simulink model "A10_DC_Motor_Antriebsstrang"  (R2017b)
settings: Solver=ode45  StartTime=0.0  StopTime=10  MaxStep=1E-3  RelTol=1e-3  EnableMultiTasking=on
values from neighbouring files (symbols this model uses):
  CM = 7.1e-7    (= 7.1e-07)    [A10_Konstanten.m]    (also in A13_Konstanten.m; A14_Konstanten.m; A16_Konstanten.m)
  JL = 2e-4    (= 0.0002)    [A10_Konstanten.m]    (also in A16_Konstanten.m)
  JR = 1.32e-6    (= 1.32e-06)    [A10_Konstanten.m]    (also in A13_Konstanten.m; A14_Konstanten.m; A16_Konstanten.m; A9_Konstanten.m = 0.004)
  KM = 38.4e-3    (= 0.0384)    [A10_Konstanten.m]    (also in A13_Konstanten.m; A14_Konstanten.m; A16_Konstanten.m)
  KN = 1/(2*pi*KM)    (= 4.14465997635)    [A10_Konstanten.m]    (also in A13_Konstanten.m; A14_Konstanten.m; A16_Konstanten.m)
  LA = 4.64e-4    (= 0.000464)    [A10_Konstanten.m]    (also in A13_Konstanten.m; A14_Konstanten.m; A16_Konstanten.m)
  MW = 0    [A10_Konstanten.m]    (also in A16_Konstanten.m = 0.001)
  R = 0.02    [A10_Konstanten.m]    (also in A13_Konstanten.m = 0.04; A14_Konstanten.m = 0.04; A16_Konstanten.m)
  RA = 4.99    [A10_Konstanten.m]    (also in A13_Konstanten.m; A14_Konstanten.m; A16_Konstanten.m)
undefined symbols (not defined in the file or in its folder): sigbuilder_block
settings Model: Creator=jbaur  LastModifiedBy=jbaur
settings DataIOCC: SaveFormat=StructureWithTime
settings OptimizationCC: ExpressionDepthLimit=2147483647  InitFltsAndDblsToZero=on  LifeSpan=inf
settings DebuggingCC: SaveWithParameterizedLinksMsg=none  SignalResolutionControl=TryResolveAllWithWarning  SolverPrmCheckMsg=warning  MultiTaskDSMMsg=warning  MultiTaskCondExecSysMsg=none  StateNameClashWarn=warning  SFUnexpectedBacktrackingDiag=warning  SFNoUnconditionalDefaultTransitionDiag=warning  SFExecutionAtInitializationDiag=none
settings HardwareCC: ProdBitPerPointer=32  ProdBitPerSizeT=32  ProdBitPerPtrDiffT=32  ProdLargestAtomicFloat=None  ProdIntDivRoundTo=Undefined  ProdEndianess=Unspecified  ProdWordSize=32  ProdHWDeviceType=32-bit Generic
settings ModelReferenceCC: PropagateSignalLabelsOutOfModel=off
settings CodeAppCC: StateflowObjectComments=on
settings GRTTargetCC: TargetFcnLib=ansi_tfl_tmw.mat  TargetLangStandard=C89/C90 (ANSI)  GeneratePreprocessorConditionals=Disable all  CombineOutputUpdateFcns=off  GRTInterface=on
settings ConfigComp: CovMetricSettings=dw  CovHtmlReporting=on  CovSaveCumulativeToWorkspaceVar=on  CovSaveSingleToWorkspaceVar=on  CovExternalEMLEnable=off  CovSFcnEnable=off

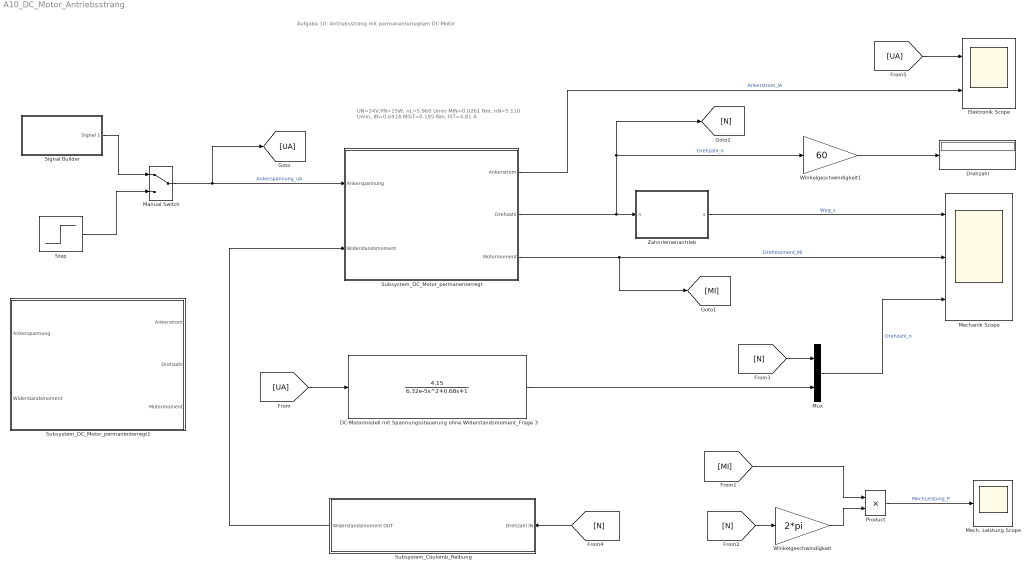
== system A10_DC_Motor_Antriebsstrang ==
  note: UN=24V,PN=15W, nL=5.960 Umin
      | MiN=0.0261 Nm, nN=5.110 Umin, IN=0.691A
      | MiST=0.185 Nm, IST=4.81 A
  note: Aufgabe 10: Antriebsstrang mit permanenterregtem DC-Motor
  DC-Motormodell mit Spannungssteuerung ohne Widerstandsmoment_Frage 3 : TransferFcn  Numerator=[4.15]  Denominator=[6.32e-5 0.68 1]
  Drehzahl : Display
  Elektronik Scope : Scope  NumInputPorts=2
  Manual Switch : ManualSwitch
  Mech. Leistung Scope : Scope
  Mechanik Scope : Scope  NumInputPorts=3
  Mux : Mux  Inputs=2
  Product : Product  RndMeth=Zero
  Signal Builder : Subsystem  Tag=STV Subsys  LoadFcn=sigbuilder_block('load');  StartFcn=sigbuilder_block('start');  StopFcn=sigbuilder_block('stop');  ClipboardFcn=sigbuilder_block('clipboard');  mask(Sigbuilder block){tuvar=[0:10]}
      mask help: Sigbuilder GUI
      mask init:
      | if ~strcmp(get_param(bdroot(gcbh),'SimulationStatus'),'stopped') tuvar = sigbuilder_block('maskInit'); end
      settings: CopyFcn=sigbuilder_block('copy');  DeleteFcn=sigbuilder_block('delete');  ModelCloseFcn=sigbuilder_block('modelClose');  PreSaveFcn=sigbuilder_block('preSave');  PauseFcn=sigbuilder_block('pause')  ContinueFcn=sigbuilder_block('continue')  NameChangeFcn=sigbuilder_block('namechange');  OpenFcn=sigbuilder_block('open',[72 61.5 772.5 424.5 ]);  CloseFcn=sigbuilder_block('close');
      mask Display: plot(0, 0, 100, 100,[2, 2, 32, 32, 2], [68, 8, 8, 68, 68],[32, 2], [38, 38], [32, 19, 2],[53, 60, 44], [32, 17, 17, 2],[16, 16, 31, 31]);txt = getActiveGroup(gcbh);text(2, 100, txt,'verticalAlignment', 'top');
  Step : Step  Time=0  After=24  SampleTime=0
  Subsystem_Coulomb_Reibung : Subsystem
  Subsystem_DC_Motor_permanenterregt : Subsystem
  Subsystem_DC_Motor_permanenterregt1 : Subsystem
  Winkelgeschwindigkeit : Gain  Gain=2*pi
  Winkelgeschwindigkeit1 : Gain  Gain=60
  Zahnriemenantrieb : Subsystem
  wires:
  Signal Builder/1(Signal 1) -> Manual Switch/1
  Step/1 -> Manual Switch/2
  Manual Switch/1 -> Subsystem_DC_Motor_permanenterregt/1(Ankerspannung), [UA]  "Ankerspannung_uA"
  Subsystem_DC_Motor_permanenterregt/1(Ankerstrom) -> Elektronik Scope/2  "Ankerstrom_iA"
  Product/1 -> Mech. Leistung Scope/1  "MechLeistung_P"
  Subsystem_Coulomb_Reibung/1(Widerstandsmoment OUT) -> Subsystem_DC_Motor_permanenterregt/2(Widerstandsmoment)
  Winkelgeschwindigkeit/1 -> Product/2
  Subsystem_DC_Motor_permanenterregt/2(Drehzahl) -> Zahnriemenantrieb/1(n), Winkelgeschwindigkeit1/1, [N]  "Drehzahl_n"
  Zahnriemenantrieb/1(s) -> Mechanik Scope/1  "Weg_s"
  Subsystem_DC_Motor_permanenterregt/3(Motormoment) -> [MI], Mechanik Scope/2  "Drehmoment_Mi"
  [MI] -> Product/1
  [N] -> Winkelgeschwindigkeit/1
  [UA] -> DC-Motormodell mit Spannungssteuerung ohne Widerstandsmoment_Frage 3/1
  Mux/1 -> Mechanik Scope/3  "Drehzahl_n"
  DC-Motormodell mit Spannungssteuerung ohne Widerstandsmoment_Frage 3/1 -> Mux/2
  [N] -> Mux/1
  [N] -> Subsystem_Coulomb_Reibung/1(Drehzahl IN)
  Winkelgeschwindigkeit1/1 -> Drehzahl/1
  [UA] -> Elektronik Scope/1

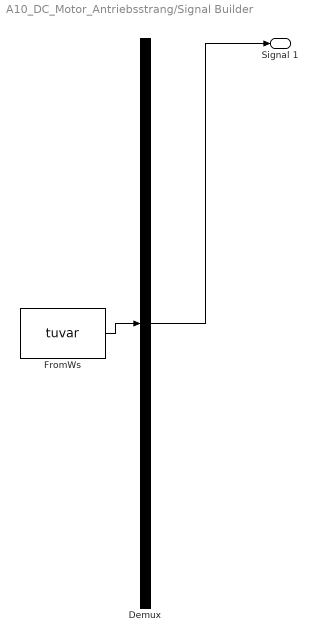
== system A10_DC_Motor_Antriebsstrang/Signal Builder ==
  Demux : Demux  Tag=STV Demux  Outputs=1
  FromWs : FromWorkspace  Tag=STV FromWs  VariableName=tuvar  SampleTime=0
      SigBuilderData=|
      | common.afterFinalStr = 'Extrapolate'
      | common.sampleTime = 0
      | dataSet.timeRange = [0 10]
      | dataSet.name = 'Group 1'
      | sbobj.Groups.Name = 'Group 1'
      | sbobj.Groups.Signals.Name = 'Signal 1'
      | sbobj.Groups.Signals.XData = [0 1 5 6 10]
      | sbobj.Groups.Signals.YData = [0 10 10 0 0]
  Signal 1 : Outport  Tag=STV Outport
  wires:
  Demux/1 -> Signal 1/1
  FromWs/1 -> Demux/1

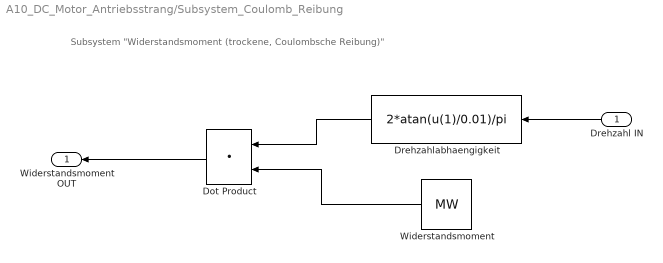
== system A10_DC_Motor_Antriebsstrang/Subsystem_Coulomb_Reibung ==
  note: Subsystem "Widerstandsmoment (trockene, Coulombsche Reibung)"
  Drehzahl IN : Inport
  Dot Product : DotProduct  InputSameDT=on  OutDataTypeStr=Inherit: Inherit via internal rule
  Drehzahlabhaengigkeit : Fcn  Expr=2*atan(u(1)/0.01)/pi
  Widerstandsmoment : Constant  Value=MW
  Widerstandsmoment OUT : Outport
  wires:
  Drehzahl IN/1 -> Drehzahlabhaengigkeit/1
  Drehzahlabhaengigkeit/1 -> Dot Product/1
  Widerstandsmoment/1 -> Dot Product/2
  Dot Product/1 -> Widerstandsmoment OUT/1

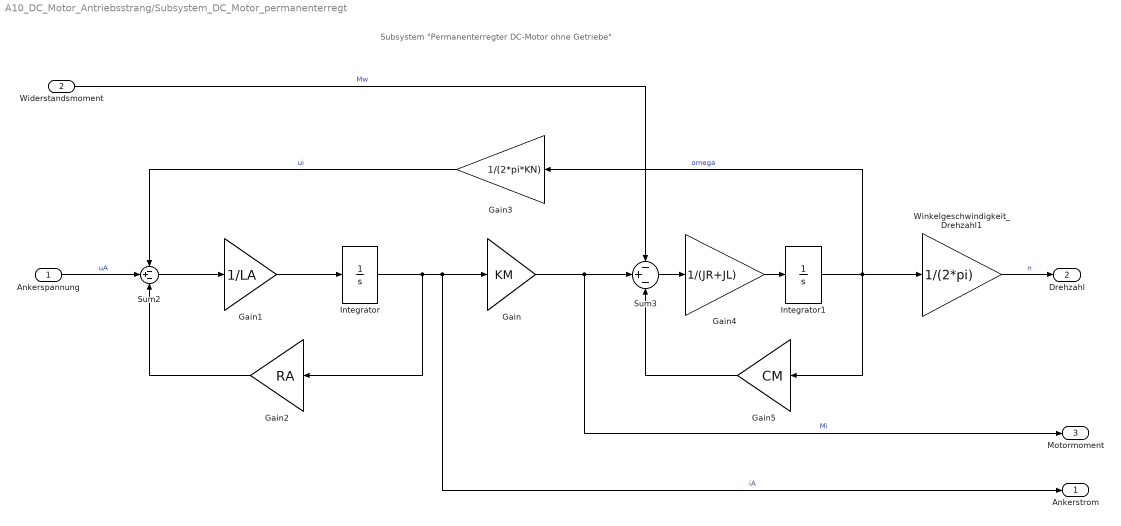
== system A10_DC_Motor_Antriebsstrang/Subsystem_DC_Motor_permanenterregt ==
  note: Subsystem "Permanenterregter DC-Motor ohne Getriebe"
  Ankerspannung : Inport
  Widerstandsmoment : Inport  Port=2
  Gain : Gain  Gain=KM
  Gain1 : Gain  Gain=1/LA
  Gain2 : Gain  Gain=RA
  Gain3 : Gain  Gain=1/(2*pi*KN)
  Gain4 : Gain  Gain=1/(JR+JL)
  Gain5 : Gain  Gain=CM
  Integrator : Integrator
  Integrator1 : Integrator
  Sum2 : Sum  Inputs=-+-
  Sum3 : Sum  Inputs=-+-
  Winkelgeschwindigkeit_Drehzahl1 : Gain  Gain=1/(2*pi)
  Ankerstrom : Outport
  Drehzahl : Outport  Port=2
  Motormoment : Outport  Port=3
  wires:
  Ankerspannung/1 -> Sum2/2  "uA"
  Gain3/1 -> Sum2/1  "ui"
  Gain/1 -> Sum3/2, Motormoment/1  "Mi"
  Winkelgeschwindigkeit_Drehzahl1/1 -> Drehzahl/1  "n"
  Sum2/1 -> Gain1/1
  Gain1/1 -> Integrator/1
  Integrator/1 -> Gain2/1, Ankerstrom/1, Gain/1  "iA"
  Sum3/1 -> Gain4/1
  Gain4/1 -> Integrator1/1
  Integrator1/1 -> Gain3/1, Winkelgeschwindigkeit_Drehzahl1/1, Gain5/1  "omega"
  Gain5/1 -> Sum3/3
  Gain2/1 -> Sum2/3
  Widerstandsmoment/1 -> Sum3/1  "Mw"

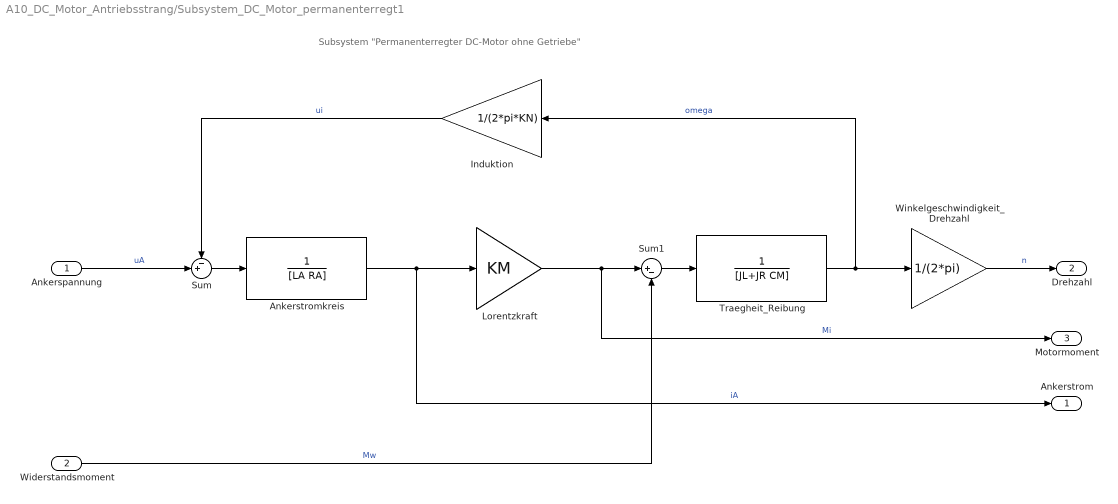
== system A10_DC_Motor_Antriebsstrang/Subsystem_DC_Motor_permanenterregt1 ==
  note: Subsystem "Permanenterregter DC-Motor ohne Getriebe"
  Ankerspannung : Inport
  Widerstandsmoment : Inport  Port=2
  Ankerstromkreis : TransferFcn  Denominator=[LA RA]
  Induktion : Gain  Gain=1/(2*pi*KN)
  Lorentzkraft : Gain  Gain=KM
  Sum : Sum  Inputs=-+|
  Sum1 : Sum  Inputs=|+-
  Traegheit_Reibung : TransferFcn  Denominator=[JL+JR CM]
  Winkelgeschwindigkeit_Drehzahl : Gain  Gain=1/(2*pi)
  Ankerstrom : Outport
  Drehzahl : Outport  Port=2
  Motormoment : Outport  Port=3
  wires:
  Ankerspannung/1 -> Sum/2  "uA"
  Sum/1 -> Ankerstromkreis/1
  Induktion/1 -> Sum/1  "ui"
  Traegheit_Reibung/1 -> Induktion/1, Winkelgeschwindigkeit_Drehzahl/1  "omega"
  Lorentzkraft/1 -> Sum1/1, Motormoment/1  "Mi"
  Sum1/1 -> Traegheit_Reibung/1
  Ankerstromkreis/1 -> Lorentzkraft/1, Ankerstrom/1  "iA"
  Widerstandsmoment/1 -> Sum1/2  "Mw"
  Winkelgeschwindigkeit_Drehzahl/1 -> Drehzahl/1  "n"

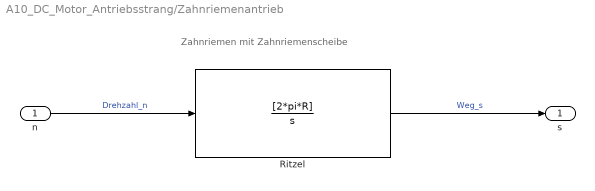
== system A10_DC_Motor_Antriebsstrang/Zahnriemenantrieb ==
  note: Zahnriemen mit Zahnriemenscheibe
  n : Inport
  Ritzel : TransferFcn  Numerator=[2*pi*R]  Denominator=[1 0]
  s : Outport
  wires:
  n/1 -> Ritzel/1  "Drehzahl_n"
  Ritzel/1 -> s/1  "Weg_s"
